simulink model "matlab model"  (R2023a)
settings: Solver=ode4  StartTime=0.0  StopTime=0.15  FixedStep=1e-6  RelTol=1e-3  EnableMultiTasking=on
libraries: neural x15, spsMosfetLib x15, simulink x10, spsMeanLib x6, spsSeriesRLCBranchLib x4, spsVoltageMeasurementLib x3, spsDCVoltageSourceLib x2, spsThreePhaseVIMeasurementLib x1, sps_lib x1
(part 2 of 2)

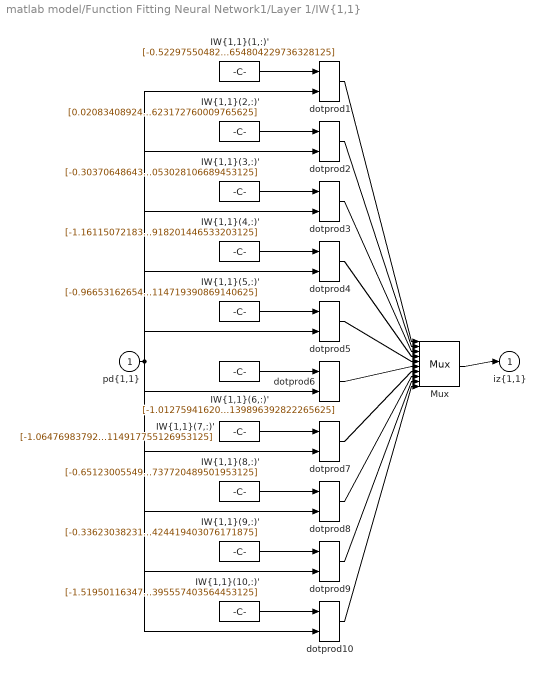
== system matlab model/Function Fitting Neural Network1/Layer 1/IW{1,1} ==
  "pd{1,1}" : Inport  PortDimensions=6
      mask Display: e = 0.06;c1 = [120 230 180]/255;c2 = ([120 230 180]+0)/(256+128);c3 = ([120 230 180]+128)/(256+128);patch([0 1 1 0],[0 0 1 1],c1);patch([0 1 1 1-e 1-e 0+e],[0 0 1 1-e 0+e 0+e],c2);patch([0 0 1 1-e 0+e 0+e],[0 1 1 1-e 1-e 0+e],c3);plot([0 1 1 0 0],[0 0 1 1 0]);
  "IW{1,1}(1,:)'" : Constant  Value=[-0.52297550482318200248954553899238817393779754638671875;1.2817116401960404470372623109142296016216278076171875;-0.87178375722353751431370483260252512991428375244140625;0.9736804156704390589283093504491262137889862060546875;0.79058075591387855229896786113386042416095733642578125;-0.092612446000115256072859892810811288654804229736328125]
      mask Display: e = 0.06;c1 = [120 150 230]/255;c2 = ([120 150 230]+0)/383;c3 = ([120 150 230]+128)/383;patch([0 1 1 0],[0 0 1 1],c1);patch([0 1 1 1-e 1-e 0+e],[0 0 1 1-e 0+e 0+e],c2);patch([0 0 1 1-e 0+e 0+e],[0 1 1 1-e 1-e 0+e],c3);plot([0 1 1 0 0],[0 0 1 1 0]);disp('Weights');
  "IW{1,1}(10,:)'" : Constant  Value=[-1.51950116347804620176020762301050126552581787109375;-0.38063341596361055518826788102160207927227020263671875;-0.50322839528787655094532738075940869748592376708984375;-0.6963550822816453322872121134423650801181793212890625;0.9256690533945246546210228189011104404926300048828125;-0.415878777312412684086240233227727003395557403564453125]
      mask Display: e = 0.06;c1 = [120 150 230]/255;c2 = ([120 150 230]+0)/383;c3 = ([120 150 230]+128)/383;patch([0 1 1 0],[0 0 1 1],c1);patch([0 1 1 1-e 1-e 0+e],[0 0 1 1-e 0+e 0+e],c2);patch([0 0 1 1-e 0+e 0+e],[0 1 1 1-e 1-e 0+e],c3);plot([0 1 1 0 0],[0 0 1 1 0]);disp('Weights');
  "IW{1,1}(2,:)'" : Constant  Value=[0.020834089246089947111695295234312652610242366790771484375;1.22438242565523491833801017492078244686126708984375;-0.285686755930494917787854092239285819232463836669921875;-1.366404366273007209287015939480625092983245849609375;-0.84787032821659169545824852320947684347629547119140625;-0.198755737737303539436339860912994481623172760009765625]
      mask Display: e = 0.06;c1 = [120 150 230]/255;c2 = ([120 150 230]+0)/383;c3 = ([120 150 230]+128)/383;patch([0 1 1 0],[0 0 1 1],c1);patch([0 1 1 1-e 1-e 0+e],[0 0 1 1-e 0+e 0+e],c2);patch([0 0 1 1-e 0+e 0+e],[0 1 1 1-e 1-e 0+e],c3);plot([0 1 1 0 0],[0 0 1 1 0]);disp('Weights');
  "IW{1,1}(3,:)'" : Constant  Value=[-0.303706486433932221213893853928311727941036224365234375;-0.038732511429090309140743642046800232492387294769287109375;-1.2446438109150228523702708116616122424602508544921875;-1.406126095391925456823400963912717998027801513671875;0.61963578275785546889409260984393768012523651123046875;-0.181941932240165915590779377453145571053028106689453125]
      mask Display: e = 0.06;c1 = [120 150 230]/255;c2 = ([120 150 230]+0)/383;c3 = ([120 150 230]+128)/383;patch([0 1 1 0],[0 0 1 1],c1);patch([0 1 1 1-e 1-e 0+e],[0 0 1 1-e 0+e 0+e],c2);patch([0 0 1 1-e 0+e 0+e],[0 1 1 1-e 1-e 0+e],c3);plot([0 1 1 0 0],[0 0 1 1 0]);disp('Weights');
  "IW{1,1}(4,:)'" : Constant  Value=[-1.1611507218378529504576590625219978392124176025390625;0.0021212588327923546059616821679583154036663472652435302734375;-1.0608023759211135939040104858577251434326171875;-0.8798328478298083066277968100621365010738372802734375;-0.74403835794904871203669927126611582934856414794921875;-0.539262202008711444278787894290871918201446533203125]
      mask Display: e = 0.06;c1 = [120 150 230]/255;c2 = ([120 150 230]+0)/383;c3 = ([120 150 230]+128)/383;patch([0 1 1 0],[0 0 1 1],c1);patch([0 1 1 1-e 1-e 0+e],[0 0 1 1-e 0+e 0+e],c2);patch([0 0 1 1-e 0+e 0+e],[0 1 1 1-e 1-e 0+e],c3);plot([0 1 1 0 0],[0 0 1 1 0]);disp('Weights');
  "IW{1,1}(5,:)'" : Constant  Value=[-0.96653162654265079023474527275539003312587738037109375;-0.56407253212853325496922707316116429865360260009765625;1.5467954910394154932617993836174719035625457763671875;0.4077396135793940334934859492932446300983428955078125;-0.385551166328934324933896959919366054236888885498046875;-0.63011397048875839033144075074233114719390869140625]
      mask Display: e = 0.06;c1 = [120 150 230]/255;c2 = ([120 150 230]+0)/383;c3 = ([120 150 230]+128)/383;patch([0 1 1 0],[0 0 1 1],c1);patch([0 1 1 1-e 1-e 0+e],[0 0 1 1-e 0+e 0+e],c2);patch([0 0 1 1-e 0+e 0+e],[0 1 1 1-e 1-e 0+e],c3);plot([0 1 1 0 0],[0 0 1 1 0]);disp('Weights');
  "IW{1,1}(6,:)'" : Constant  Value=[-1.0127594162033537461553578395978547632694244384765625;1.1239124206940236394558496613171882927417755126953125;1.184355543413506239858179469592869281768798828125;0.62233663680027462294930273856152780354022979736328125;0.355744339420696442655156488399370573461055755615234375;0.025405103035661714960813384323046193458139896392822265625]
      mask Display: e = 0.06;c1 = [120 150 230]/255;c2 = ([120 150 230]+0)/383;c3 = ([120 150 230]+128)/383;patch([0 1 1 0],[0 0 1 1],c1);patch([0 1 1 1-e 1-e 0+e],[0 0 1 1-e 0+e 0+e],c2);patch([0 0 1 1-e 0+e 0+e],[0 1 1 1-e 1-e 0+e],c3);plot([0 1 1 0 0],[0 0 1 1 0]);disp('Weights');
  "IW{1,1}(7,:)'" : Constant  Value=[-1.064769837929170126500366677646525204181671142578125;-0.371155648377578806229593055832083337008953094482421875;0.3313678427849782170966363992192782461643218994140625;0.53032790908555382802802569131017662584781646728515625;1.0161426234237185273201475865789689123630523681640625;1.2993598773377375010795731213875114917755126953125]
      mask Display: e = 0.06;c1 = [120 150 230]/255;c2 = ([120 150 230]+0)/383;c3 = ([120 150 230]+128)/383;patch([0 1 1 0],[0 0 1 1],c1);patch([0 1 1 1-e 1-e 0+e],[0 0 1 1-e 0+e 0+e],c2);patch([0 0 1 1-e 0+e 0+e],[0 1 1 1-e 1-e 0+e],c3);plot([0 1 1 0 0],[0 0 1 1 0]);disp('Weights');
  "IW{1,1}(8,:)'" : Constant  Value=[-0.65123005549075141384918197218212299048900604248046875;-0.97020952051313480435368319376721046864986419677734375;-1.1082373678875534483978526623104698956012725830078125;-0.12429678378193796672857018847935250960290431976318359375;-1.0389191803820729820273527366225607693195343017578125;0.73438223954719294983561894696322269737720489501953125]
      mask Display: e = 0.06;c1 = [120 150 230]/255;c2 = ([120 150 230]+0)/383;c3 = ([120 150 230]+128)/383;patch([0 1 1 0],[0 0 1 1],c1);patch([0 1 1 1-e 1-e 0+e],[0 0 1 1-e 0+e 0+e],c2);patch([0 0 1 1-e 0+e 0+e],[0 1 1 1-e 1-e 0+e],c3);plot([0 1 1 0 0],[0 0 1 1 0]);disp('Weights');
  "IW{1,1}(9,:)'" : Constant  Value=[-0.336230382311246189797060424098162911832332611083984375;0.85532713338638555189419321322930045425891876220703125;-0.9633929790872717280336701151099987328052520751953125;0.1600857103973878092784133286841097287833690643310546875;1.3549634524833036319790835477760992944240570068359375;1.0798219373778195073754204713623039424419403076171875]
      mask Display: e = 0.06;c1 = [120 150 230]/255;c2 = ([120 150 230]+0)/383;c3 = ([120 150 230]+128)/383;patch([0 1 1 0],[0 0 1 1],c1);patch([0 1 1 1-e 1-e 0+e],[0 0 1 1-e 0+e 0+e],c2);patch([0 0 1 1-e 0+e 0+e],[0 1 1 1-e 1-e 0+e],c3);plot([0 1 1 0 0],[0 0 1 1 0]);disp('Weights');
  Mux : Mux  Inputs=10
      mask Display: e = 0.06;c1 = [120 150 230]/255;c2 = ([120 150 230]+0)/383;c3 = ([120 150 230]+128)/383;patch([0 1 1 0],[0 0 1 1],c1);patch([0 1 1 1-e 1-e 0+e],[0 0 1 1-e 0+e 0+e],c2);patch([0 0 1 1-e 0+e 0+e],[0 1 1 1-e 1-e 0+e],c3);plot([0 1 1 0 0],[0 0 1 1 0]);disp('Mux');
  dotprod{1..10} (10 alike) : neural/Weight Functions/dotprod
  "iz{1,1}" : Outport
      mask Display: e = 0.06;c1 = [120 230 180]/255;c2 = ([120 230 180]+0)/(256+128);c3 = ([120 230 180]+128)/(256+128);patch([0 1 1 0],[0 0 1 1],c1);patch([0 1 1 1-e 1-e 0+e],[0 0 1 1-e 0+e 0+e],c2);patch([0 0 1 1-e 0+e 0+e],[0 1 1 1-e 1-e 0+e],c3);plot([0 1 1 0 0],[0 0 1 1 0]);
  wires:
  "IW{1,1}(1,:)'"/1 -> dotprod1/1
  "pd{1,1}"/1 -> dotprod1/2, dotprod2/2, dotprod3/2, dotprod4/2, dotprod5/2, dotprod6/2, dotprod7/2, dotprod8/2, dotprod9/2, dotprod10/2
  dotprod1/1 -> Mux/1
  "IW{1,1}(2,:)'"/1 -> dotprod2/1
  dotprod2/1 -> Mux/2
  "IW{1,1}(3,:)'"/1 -> dotprod3/1
  dotprod3/1 -> Mux/3
  "IW{1,1}(4,:)'"/1 -> dotprod4/1
  dotprod4/1 -> Mux/4
  "IW{1,1}(5,:)'"/1 -> dotprod5/1
  dotprod5/1 -> Mux/5
  "IW{1,1}(6,:)'"/1 -> dotprod6/1
  dotprod6/1 -> Mux/6
  "IW{1,1}(7,:)'"/1 -> dotprod7/1
  dotprod7/1 -> Mux/7
  "IW{1,1}(8,:)'"/1 -> dotprod8/1
  dotprod8/1 -> Mux/8
  "IW{1,1}(9,:)'"/1 -> dotprod9/1
  dotprod9/1 -> Mux/9
  "IW{1,1}(10,:)'"/1 -> dotprod10/1
  dotprod10/1 -> Mux/10
  Mux/1 -> "iz{1,1}"/1

== system matlab model/Function Fitting Neural Network1/Layer 2/Delays 1 ==
  "p{2}" : Inport  PortDimensions=10
      mask Display: e = 0.06;c1 = [120 230 180]/255;c2 = ([120 230 180]+0)/(256+128);c3 = ([120 230 180]+128)/(256+128);patch([0 1 1 0],[0 0 1 1],c1);patch([0 1 1 1-e 1-e 0+e],[0 0 1 1-e 0+e 0+e],c2);patch([0 0 1 1-e 0+e 0+e],[0 1 1 1-e 1-e 0+e],c3);plot([0 1 1 0 0],[0 0 1 1 0]);
  mux : Mux  Inputs=1
      mask Display: e = 0.06;c1 = [120 150 230]/255;c2 = ([120 150 230]+0)/383;c3 = ([120 150 230]+128)/383;patch([0 1 1 0],[0 0 1 1],c1);patch([0 1 1 1-e 1-e 0+e],[0 0 1 1-e 0+e 0+e],c2);patch([0 0 1 1-e 0+e 0+e],[0 1 1 1-e 1-e 0+e],c3);plot([0 1 1 0 0],[0 0 1 1 0]);disp('Mux')
  "pd{2,1}" : Outport
      mask Display: e = 0.06;c1 = [120 230 180]/255;c2 = ([120 230 180]+0)/(256+128);c3 = ([120 230 180]+128)/(256+128);patch([0 1 1 0],[0 0 1 1],c1);patch([0 1 1 1-e 1-e 0+e],[0 0 1 1-e 0+e 0+e],c2);patch([0 0 1 1-e 0+e 0+e],[0 1 1 1-e 1-e 0+e],c3);plot([0 1 1 0 0],[0 0 1 1 0]);
  wires:
  "p{2}"/1 -> mux/1
  mux/1 -> "pd{2,1}"/1

== system matlab model/Function Fitting Neural Network1/Layer 2/LW{2,1} ==
  "ad{2,1}" : Inport  PortDimensions=10
      mask Display: e = 0.06;c1 = [120 230 180]/255;c2 = ([120 230 180]+0)/(256+128);c3 = ([120 230 180]+128)/(256+128);patch([0 1 1 0],[0 0 1 1],c1);patch([0 1 1 1-e 1-e 0+e],[0 0 1 1-e 0+e 0+e],c2);patch([0 0 1 1-e 0+e 0+e],[0 1 1 1-e 1-e 0+e],c3);plot([0 1 1 0 0],[0 0 1 1 0]);
  "IW{2,1}(1,:)'" : Constant  Value=[0.73867454900789464300459030710044316947460174560546875;-0.08704065207198065368121575602344819344580173492431640625;0.52408937818549905518494824718800373375415802001953125;0.81850809770628696337979590680333785712718963623046875;0.311711683272173856185105478289187885820865631103515625;-0.1454256869371632898690904767136089503765106201171875;-0.65652281621186714399840411715558730065822601318359375;0.08706942896730753000955616016653948463499546051025390625;-0.346474401256624597866817794056260026991367340087890625;-0.466892195860454550793150474419235251843929290771484375]
      mask Display: e = 0.06;c1 = [120 150 230]/255;c2 = ([120 150 230]+0)/383;c3 = ([120 150 230]+128)/383;patch([0 1 1 0],[0 0 1 1],c1);patch([0 1 1 1-e 1-e 0+e],[0 0 1 1-e 0+e 0+e],c2);patch([0 0 1 1-e 0+e 0+e],[0 1 1 1-e 1-e 0+e],c3);plot([0 1 1 0 0],[0 0 1 1 0]);disp('weights');
  Mux : Mux  Inputs=1
      mask Display: e = 0.06;c1 = [120 150 230]/255;c2 = ([120 150 230]+0)/383;c3 = ([120 150 230]+128)/383;patch([0 1 1 0],[0 0 1 1],c1);patch([0 1 1 1-e 1-e 0+e],[0 0 1 1-e 0+e 0+e],c2);patch([0 0 1 1-e 0+e 0+e],[0 1 1 1-e 1-e 0+e],c3);plot([0 1 1 0 0],[0 0 1 1 0]);disp('Mux');
  dotprod1 : neural/Weight Functions/dotprod
  "lz{2,1}" : Outport
      mask Display: e = 0.06;c1 = [120 230 180]/255;c2 = ([120 230 180]+0)/(256+128);c3 = ([120 230 180]+128)/(256+128);patch([0 1 1 0],[0 0 1 1],c1);patch([0 1 1 1-e 1-e 0+e],[0 0 1 1-e 0+e 0+e],c2);patch([0 0 1 1-e 0+e 0+e],[0 1 1 1-e 1-e 0+e],c3);plot([0 1 1 0 0],[0 0 1 1 0]);
  wires:
  "IW{2,1}(1,:)'"/1 -> dotprod1/1
  "ad{2,1}"/1 -> dotprod1/2
  dotprod1/1 -> Mux/1
  Mux/1 -> "lz{2,1}"/1

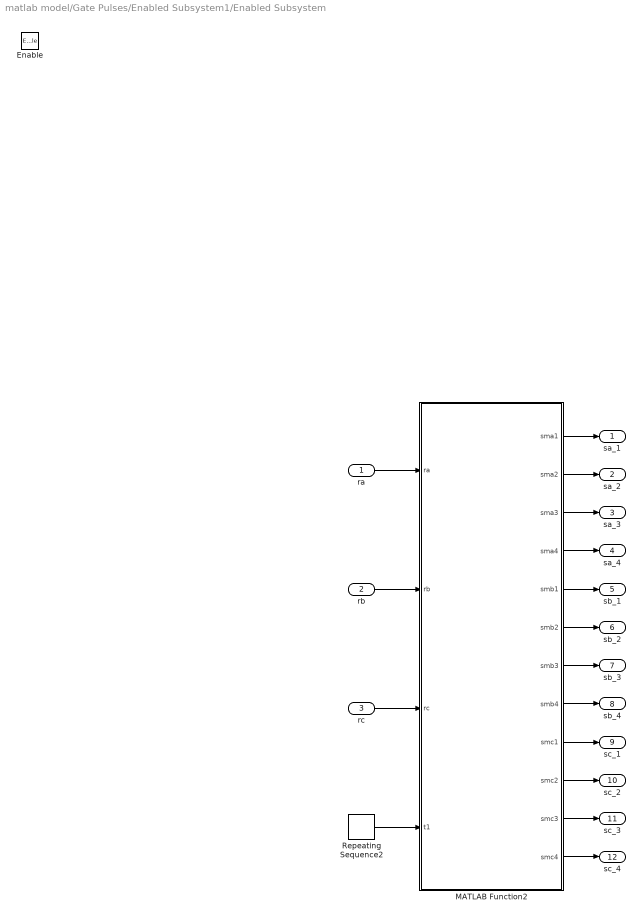
== system matlab model/Gate Pulses/Enabled Subsystem1/Enabled Subsystem ==
  ra : Inport
  rb : Inport  Port=2
  rc : Inport  Port=3
  Enable : EnablePort
  MATLAB Function2 : MATLAB Function  TreatAsAtomicUnit=on
  Repeating Sequence2 : simulink/Sources/Repeating Sequence  rep_seq_t=[0 1/2000 1/1000]  rep_seq_y=[-1 1 -1]
  sa_1 : Outport  VectorParamsAs1DForOutWhenUnconnected=off
  sa_2 : Outport  Port=2  VectorParamsAs1DForOutWhenUnconnected=off
  sa_3 : Outport  Port=3  VectorParamsAs1DForOutWhenUnconnected=off
  sa_4 : Outport  Port=4  VectorParamsAs1DForOutWhenUnconnected=off
  sb_1 : Outport  Port=5  VectorParamsAs1DForOutWhenUnconnected=off
  sb_2 : Outport  Port=6  VectorParamsAs1DForOutWhenUnconnected=off
  sb_3 : Outport  Port=7  VectorParamsAs1DForOutWhenUnconnected=off
  sb_4 : Outport  Port=8  VectorParamsAs1DForOutWhenUnconnected=off
  sc_1 : Outport  Port=9  VectorParamsAs1DForOutWhenUnconnected=off
  sc_2 : Outport  Port=10  VectorParamsAs1DForOutWhenUnconnected=off
  sc_3 : Outport  Port=11  VectorParamsAs1DForOutWhenUnconnected=off
  sc_4 : Outport  Port=12  VectorParamsAs1DForOutWhenUnconnected=off
  wires:
  MATLAB Function2/12(smc4) -> sc_4/1
  MATLAB Function2/11(smc3) -> sc_3/1
  MATLAB Function2/10(smc2) -> sc_2/1
  MATLAB Function2/9(smc1) -> sc_1/1
  MATLAB Function2/8(smb4) -> sb_4/1
  MATLAB Function2/7(smb3) -> sb_3/1
  MATLAB Function2/6(smb2) -> sb_2/1
  MATLAB Function2/5(smb1) -> sb_1/1
  MATLAB Function2/4(sma4) -> sa_4/1
  MATLAB Function2/3(sma3) -> sa_3/1
  MATLAB Function2/2(sma2) -> sa_2/1
  MATLAB Function2/1(sma1) -> sa_1/1
  rc/1 -> MATLAB Function2/3(rc)
  rb/1 -> MATLAB Function2/2(rb)
  ra/1 -> MATLAB Function2/1(ra)
  Repeating Sequence2/1 -> MATLAB Function2/4(t1)

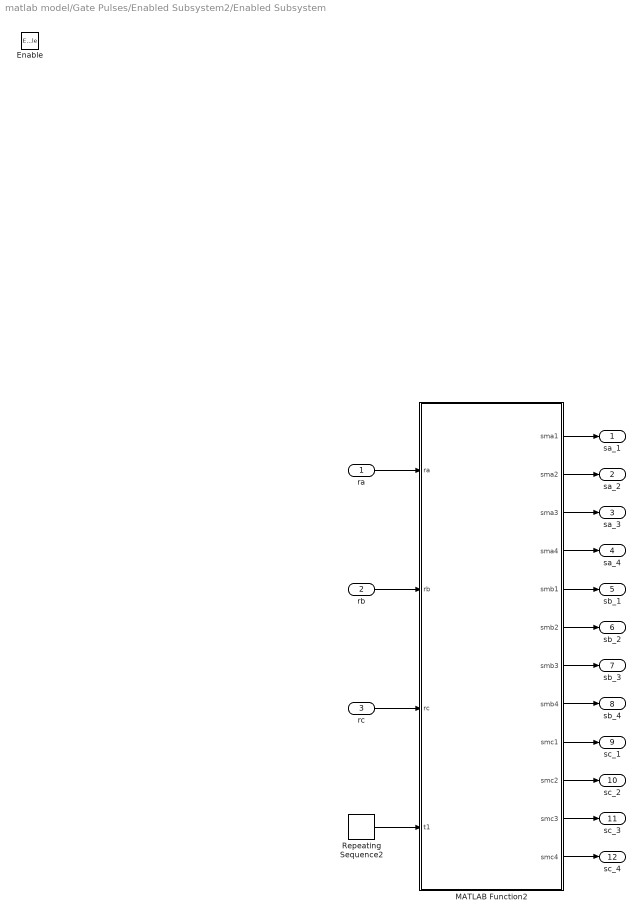
== system matlab model/Gate Pulses/Enabled Subsystem2/Enabled Subsystem ==
  ra : Inport
  rb : Inport  Port=2
  rc : Inport  Port=3
  Enable : EnablePort
  MATLAB Function2 : MATLAB Function  TreatAsAtomicUnit=on
  Repeating Sequence2 : simulink/Sources/Repeating Sequence  rep_seq_t=[0 1/2000 1/1000]  rep_seq_y=[-1 1 -1]
  sa_1 : Outport  VectorParamsAs1DForOutWhenUnconnected=off
  sa_2 : Outport  Port=2  VectorParamsAs1DForOutWhenUnconnected=off
  sa_3 : Outport  Port=3  VectorParamsAs1DForOutWhenUnconnected=off
  sa_4 : Outport  Port=4  VectorParamsAs1DForOutWhenUnconnected=off
  sb_1 : Outport  Port=5  VectorParamsAs1DForOutWhenUnconnected=off
  sb_2 : Outport  Port=6  VectorParamsAs1DForOutWhenUnconnected=off
  sb_3 : Outport  Port=7  VectorParamsAs1DForOutWhenUnconnected=off
  sb_4 : Outport  Port=8  VectorParamsAs1DForOutWhenUnconnected=off
  sc_1 : Outport  Port=9  VectorParamsAs1DForOutWhenUnconnected=off
  sc_2 : Outport  Port=10  VectorParamsAs1DForOutWhenUnconnected=off
  sc_3 : Outport  Port=11  VectorParamsAs1DForOutWhenUnconnected=off
  sc_4 : Outport  Port=12  VectorParamsAs1DForOutWhenUnconnected=off
  wires:
  Repeating Sequence2/1 -> MATLAB Function2/4(t1)
  ra/1 -> MATLAB Function2/1(ra)
  rb/1 -> MATLAB Function2/2(rb)
  rc/1 -> MATLAB Function2/3(rc)
  MATLAB Function2/1(sma1) -> sa_1/1
  MATLAB Function2/2(sma2) -> sa_2/1
  MATLAB Function2/3(sma3) -> sa_3/1
  MATLAB Function2/4(sma4) -> sa_4/1
  MATLAB Function2/5(smb1) -> sb_1/1
  MATLAB Function2/6(smb2) -> sb_2/1
  MATLAB Function2/7(smb3) -> sb_3/1
  MATLAB Function2/8(smb4) -> sb_4/1
  MATLAB Function2/9(smc1) -> sc_1/1
  MATLAB Function2/10(smc2) -> sc_2/1
  MATLAB Function2/11(smc3) -> sc_3/1
  MATLAB Function2/12(smc4) -> sc_4/1

== system matlab model/Subsystem/Enabled Subsystem/Subsystem ==
  f1 : Inport
  f2 : Inport  Port=2
  sa1 : Inport  Port=3
  sa2 : Inport  Port=4
  sb1 : Inport  Port=5
  sb2 : Inport  Port=6
  sc1 : Inport  Port=7
  sc2 : Inport  Port=8
  MATLAB Function : MATLAB Function  TreatAsAtomicUnit=on
  a1 : Outport  VectorParamsAs1DForOutWhenUnconnected=off
  a2 : Outport  Port=2  VectorParamsAs1DForOutWhenUnconnected=off
  b1 : Outport  Port=3  VectorParamsAs1DForOutWhenUnconnected=off
  b2 : Outport  Port=4  VectorParamsAs1DForOutWhenUnconnected=off
  c1 : Outport  Port=5  VectorParamsAs1DForOutWhenUnconnected=off
  c2 : Outport  Port=6  VectorParamsAs1DForOutWhenUnconnected=off
  wires:
  MATLAB Function/6(c2) -> c2/1
  MATLAB Function/5(c1) -> c1/1
  MATLAB Function/4(b2) -> b2/1
  MATLAB Function/3(b1) -> b1/1
  MATLAB Function/1(a1) -> a1/1
  MATLAB Function/2(a2) -> a2/1
  f1/1 -> MATLAB Function/1(f1)
  f2/1 -> MATLAB Function/2(f2)
  sa1/1 -> MATLAB Function/3(sa1)
  sa2/1 -> MATLAB Function/4(sa2)
  sb1/1 -> MATLAB Function/5(sb1)
  sb2/1 -> MATLAB Function/6(sb2)
  sc1/1 -> MATLAB Function/7(sc1)
  sc2/1 -> MATLAB Function/8(sc2)

== matlab function matlab model/Gate Pulses/Enabled Subsystem2/Enabled Subsystem/MATLAB Function2 ==
  data: sma1 output; sma2 output; sma3 output; sma4 output; smb1 output; smb2 output; smb3 output; smb4 output; smc1 output; smc2 output; ra input; rb input; rc input; t1 input; smc3 output; smc4 output
function [sma1,sma2,sma3, sma4, smb1,smb2,smb3,smb4,smc1,smc2,smc3,smc4] = fcn(ra,rb,rc,t1)
%#codegen
if(ra>=t1)
    sma1=1;
    sma2=0;
    sma3=1;
    sma4=0;
else
    sma1=0;
    sma2=0;
    sma3=0;
    sma4=1; 
end
if(rb>=t1)
    smb1=1;
    smb2=0;
    smb3=1;
    smb4=0;
else
    smb1=0;
    smb2=0;
    smb3=0;
    smb4=1; 
end
if(rc>=t1)
    smc1=1;
    smc2=0;
    smc3=1;
    smc4=0;
else
    smc1=0;
    smc2=0;
    smc3=0;
    smc4=1; 
end
end

== matlab function matlab model/Gate Pulses/Subsystem2/MATLAB Function1 ==
  data: a2 input; y output; b2 input; c2 input
function y = fcn(a2,b2,c2)
%#codegen
if(a2==b2==c2)
    y=1;
else
    y=0;
end

== matlab function matlab model/Gate Pulses/Enabled Subsystem1/Enabled Subsystem/MATLAB Function2 ==
  data: sma1 output; sma2 output; sma3 output; sma4 output; smb1 output; smb2 output; smb3 output; smb4 output; smc1 output; smc2 output; ra input; rb input; rc input; t1 input; smc3 output; smc4 output
function [sma1,sma2,sma3, sma4, smb1,smb2,smb3,smb4,smc1,smc2,smc3,smc4] = fcn(ra,rb,rc,t1)
%#codegen
if(ra>=t1)
    sma1=0;
    sma2=1;
    sma3=1;
    sma4=0;
else
    sma1=0;
    sma2=0;
    sma3=0;
    sma4=1; 
end
if(rb>=t1)
    smb1=0;
    smb2=1;
    smb3=1;
    smb4=0;
else
    smb1=0;
    smb2=0;
    smb3=0;
    smb4=1; 
end
if(rc>=t1)
    smc1=0;
    smc2=1;
    smc3=1;
    smc4=0;
else
    smc1=0;
    smc2=0;
    smc3=0;
    smc4=1; 
end
end

== matlab function matlab model/Gate Pulses/MATLAB Function ==
  data: ra input; sa1 output; rb input; rc input; t1 input; t2 input; sa2 output; sa3 output; sa4 output; sb1 output; sb2 output; sb3 output; sb4 output; sc1 output; sc2 output; sc3 output; sc4 output
function [sa1,sa2,sa3,sa4,sb1,sb2,sb3,sb4,sc1,sc2,sc3,sc4] = fcn(ra,rb,rc,t1,t2)
%#codegen
if(ra>=t1)
    sa1=1;
    sa2=0;
    sa3=1;
    sa4=0;
elseif(ra<t1&&ra>t2)
    sa1=0;
    sa2=1;
    sa3=1;
    sa4=0;
else
    sa1=0;
    sa2=0;
    sa3=0;
    sa4=1;
end
if(rb>=t1)
    sb1=1;
    sb2=0;
    sb3=1;
    sb4=0;
elseif(rb<t1&&rb>t2)
    sb1=0;
    sb2=1;
    sb3=1;
    sb4=0;
else
    sb1=0;
    sb2=0;
    sb3=0;
    sb4=1;
end
if(rc>=t1)
    sc1=1;
    sc2=0;
    sc3=1;
    sc4=0;
elseif(rc<t1&&rc>t2)
    sc1=0;
    sc2=1;
    sc3=1;
    sc4=0;
else
    sc1=0;
    sc2=0;
    sc3=0;
    sc4=1;
end

== matlab function matlab model/Gate Pulses/Subsystem1/MATLAB Function1 ==
  data: a2 input; y output; b2 input; c2 input
function y = fcn(a2,b2,c2)
%#codegen
if(a2==b2==c2)
    y=1;
else
    y=0;
end

== matlab function matlab model/Subsystem/Enabled Subsystem/Subsystem/MATLAB Function ==
  data: f1 input; a1 output; f2 input; sa1 input; sa2 input; sb1 input; sb2 input; sc1 input; sc2 input; a2 output; b1 output; b2 output; c1 output; c2 output
function [a1,a2,b1,b2,c1,c2] = fcn(f1,f2,sa1,sa2,sb1,sb2,sc1,sc2)
%#codegen
a1=1;
a2=1;
b1=1;
b2=1;
c1=1;
c2=1;
if(f1==1&&f2==1)
    a1=1;
    a2=1;
    b1=1;
    b2=1;
    c1=1;
    c2=1;
else
    if(f2==1)
     if(sa1==0)
            a1=0;
            a2=1;
            b1=1;
            b2=1;
            c1=1;
            c2=1;
     end
     if(sb1==0)
            a1=1;
            a2=1;
            b1=0;
            b2=1;
            c1=1;
            c2=1;
     end
     if(sc1==0)
            a1=1;
            a2=1;
            b1=1;
            b2=1;
            c1=0;
            c2=1;
     end
    else
      if(sa2==0)
            a1=1;
            a2=0;
            b1=1;
            b2=1;
            c1=1;
            c2=1;
     end
     if(sb2==0)
            a1=1;
            a2=1;
            b1=1;
            b2=0;
            c1=1;
            c2=1;
     end
     if(sc2==0)
            a1=1;
            a2=1;
            b1=1;
            b2=1;
            c1=1;
            c2=0;
     end       
    end
end
